simulink model "Simulaciones"  (R2023a)
settings: Solver=ode23s  StartTime=0.0  StopTime=2000  RelTol=1e-3
settings Model: Creator=franc  LastModifiedBy=Ricardo Pérez

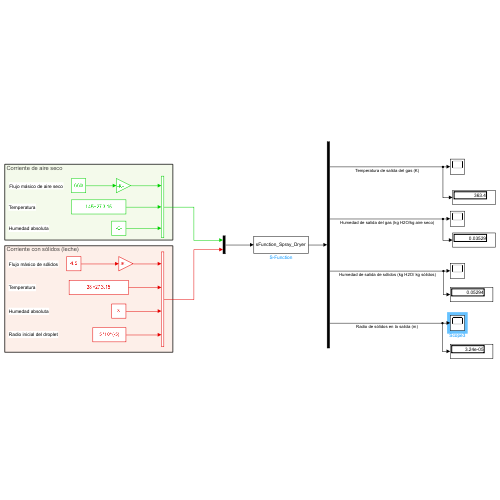
[thumbnail: Simulink's stored preview of the top-level diagram]
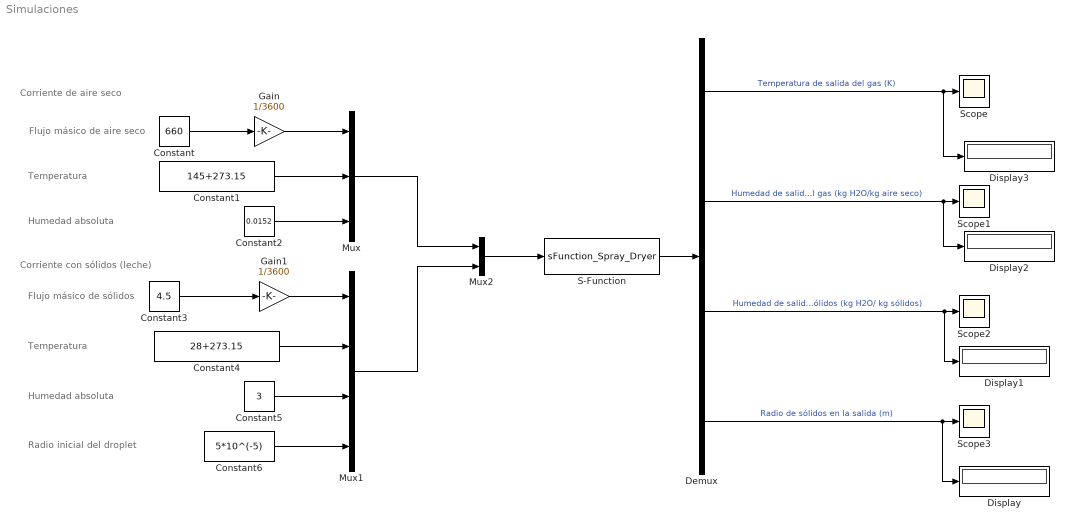
== system Simulaciones ==
  note: Flujo másico de aire seco
  note: Corriente de aire seco
  note: Corriente con sólidos (leche)
  note: Temperatura
  note: Humedad absoluta
  note: Flujo másico de sólidos
  note: Temperatura
  note: Humedad absoluta
  note: Radio inicial del droplet
  Constant : Constant  Value=660
  Constant1 : Constant  Value=145+273.15
  Constant2 : Constant  Value=0.0152
  Constant3 : Constant  Value=4.5
  Constant4 : Constant  Value=28+273.15
  Constant5 : Constant  Value=3
  Constant6 : Constant  Value=5*10^(-5)
  Demux : Demux
  Display{,1..3} (4 alike) : Display
  Gain : Gain  Gain=1/3600
  Gain1 : Gain  Gain=1/3600
  Mux : Mux  Inputs=3
  Mux1 : Mux
  Mux2 : Mux  Inputs=2
  S-Function : S-Function  FunctionName=sFunction_Spray_Dryer  SFunctionDeploymentMode=off  EnableBusSupport=off
  Scope{,1..3} (4 alike) : Scope
  wires:
  Constant/1 -> Gain/1
  Constant1/1 -> Mux/2
  Constant2/1 -> Mux/3
  Constant3/1 -> Gain1/1
  Constant5/1 -> Mux1/3
  Constant4/1 -> Mux1/2
  Mux/1 -> Mux2/1
  Mux1/1 -> Mux2/2
  Mux2/1 -> S-Function/1
  Gain/1 -> Mux/1
  Gain1/1 -> Mux1/1
  S-Function/1 -> Demux/1
  Demux/1 -> Display3/1, Scope/1  "Temperatura de salida del gas (K)"
  Demux/2 -> Display2/1, Scope1/1  "Humedad de salida del gas (kg H2O/kg aire seco)"
  Demux/3 -> Display1/1, Scope2/1  "Humedad de salida de sólidos (kg H2O/ kg sólidos)"
  Demux/4 -> Display/1, Scope3/1  "Radio de sólidos en la salida (m)"
  Constant6/1 -> Mux1/4
